simulink model "IdentifikaceModeluSISO"  (Simulink 7.8)
settings: Solver=ode45  StartTime=0.0  StopTime=7500  RelTol=1e-3
undefined symbols (not defined in the file): sfunxy2
libraries: simulink x2
settings Model: Creator=frdu0449  LastModifiedBy=KRP

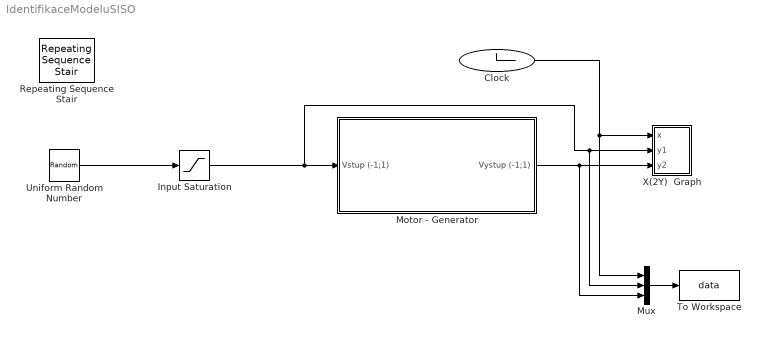
== system IdentifikaceModeluSISO ==
  Clock : Clock
  Input Saturation : Saturate  UpperLimit=1  LowerLimit=-1
  Motor - Generator : Subsystem
  Mux : Mux  Inputs=3
  Repeating Sequence Stair : simulink/Sources/Repeating Sequence Stair  OutValues=[0.8 -0.6 0.4 0.9 -0.3 -0.7 0.7 -1].'  tsamp=20  OutMin=[]  OutMax=[]  OutDataTypeStr=double  OutputDataTypeScalingMode=double  OutDataType=fixdt(0,8)  ConRadixGroup=Best Precision: Vector-wise  OutScaling=2^-12
  To Workspace : ToWorkspace  VariableName=data  SampleTime=0.25  SaveFormat=Structure
  Uniform Random Number : UniformRandomNumber  Minimum=-1.2  Maximum=1.2  Seed=615482  SampleTime=15
  X(2Y)  Graph : Subsystem  LoadFcn=sfunxy2([],[],[],'LoadBlock')  StartFcn=sfunxy2([],[],[],'Start')  StopFcn=sfunxy2([],[],[],'Stop')  mask(X(2Y) scope.){xmin=0, xmax=5, ymin=-1, ymax=1, st=-1}
      mask prompts: xmin "x-min:"; xmax "x-max:"; ymin "y-min:"; ymax "y-max:"; st "Sample time:"
      mask help: X(2Y) scope using MATLAB graph window. First input is used as time base. Enter plotting ranges.
      settings: CopyFcn=sfunxy2([],[],[],'CopyBlock')  DeleteFcn=sfunxy2([],[],[],'DeleteBlock')  NameChangeFcn=sfunxy2([],[],[],'NameChange')
      mask Help: This block can be used to explore limit cycles. Look at function sfunxy.m to see how it works.
      mask Display: plot([.05 .95 .95 .05 .05],[.45 .45 .95 .95 .45], 0.5+cos(0:0.1:2*pi)*0.3,0.7+sin(0:0.1:2*pi)*0.2)
  wires:
  Motor - Generator/1(Vystup (-1;1)) -> X(2Y)  Graph/3(y2), Mux/3
  Clock/1 -> X(2Y)  Graph/1(x), Mux/1
  Mux/1 -> To Workspace/1
  Input Saturation/1 -> Motor - Generator/1(Vstup (-1;1)), X(2Y)  Graph/2(y1), Mux/2
  Uniform Random Number/1 -> Input Saturation/1

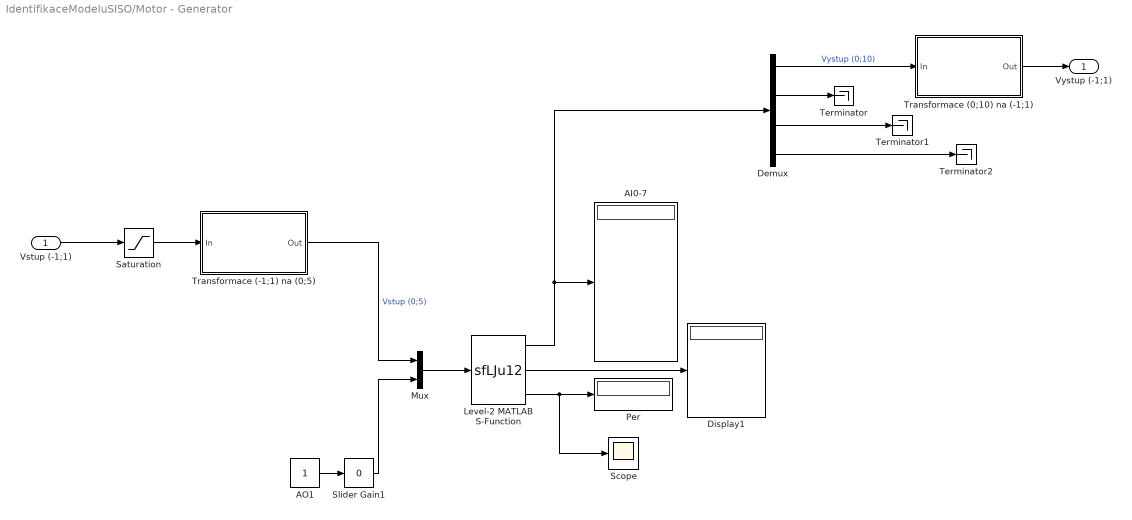
== system IdentifikaceModeluSISO/Motor - Generator ==
  Vstup (-1;1) : Inport
  AI0-7 : Display
  AO1 : Constant
  Demux : Demux
  Display1 : Display
  Level-2 MATLAB S-Function : M-S-Function  FunctionName=sfLJu12  Parameters=0,0.1,0,[0,1,2,3],[0,0,0,0]
  Mux : Mux  Inputs=2
  Per : Display
  Saturation : Saturate  UpperLimit=1  LowerLimit=-1
  Scope : Scope
      settings: YMin=0.075  YMax=0.3
  Slider Gain1 : simulink/Math Operations/Slider Gain  low=0  gain=0  high=5
  Terminator : Terminator
  Terminator1 : Terminator
  Terminator2 : Terminator
  Transformace (-1;1) na (0;5) : Subsystem
  Transformace (0;10) na (-1;1) : Subsystem
  Vystup (-1;1) : Outport
  wires:
  Mux/1 -> Level-2 MATLAB S-Function/1
  AO1/1 -> Slider Gain1/1
  Level-2 MATLAB S-Function/3 -> Per/1, Scope/1
  Level-2 MATLAB S-Function/1 -> AI0-7/1, Demux/1
  Level-2 MATLAB S-Function/2 -> Display1/1
  Vstup (-1;1)/1 -> Saturation/1
  Slider Gain1/1 -> Mux/2
  Transformace (-1;1) na (0;5)/1(Out) -> Mux/1  "Vstup (0;5)"
  Demux/2 -> Terminator/1
  Demux/3 -> Terminator1/1
  Demux/4 -> Terminator2/1
  Demux/1 -> Transformace (0;10) na (-1;1)/1(In)  "Vystup (0;10)"
  Transformace (0;10) na (-1;1)/1(Out) -> Vystup (-1;1)/1
  Saturation/1 -> Transformace (-1;1) na (0;5)/1(In)

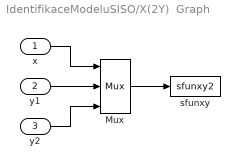
== system IdentifikaceModeluSISO/X(2Y)  Graph ==
  x : Inport
  y1 : Inport  Port=2
  y2 : Inport  Port=3
  Mux : Mux  Inputs=3
  sfunxy : S-Function  FunctionName=sfunxy2  Parameters=[xmin xmax ymin ymax], st  EnableBusSupport=off
  wires:
  y2/1 -> Mux/3
  y1/1 -> Mux/2
  x/1 -> Mux/1
  Mux/1 -> sfunxy/1

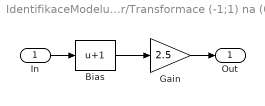
== system IdentifikaceModeluSISO/Motor - Generator/Transformace (-1;1) na (0;5) ==
  In : Inport
  Bias : Bias  Bias=1
  Gain : Gain  Gain=2.5
  Out : Outport
  wires:
  Bias/1 -> Gain/1
  In/1 -> Bias/1
  Gain/1 -> Out/1

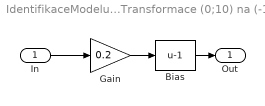
== system IdentifikaceModeluSISO/Motor - Generator/Transformace (0;10) na (-1;1) ==
  In : Inport
  Bias : Bias  Bias=-1
  Gain : Gain  Gain=0.2
  Out : Outport
  wires:
  Gain/1 -> Bias/1
  In/1 -> Gain/1
  Bias/1 -> Out/1
